simulink model "LQR_control_2019b"  (R2021a)
settings: Solver=VariableStepAuto  StartTime=0.0  StopTime=10.0  RelTol=1e-3
undefined symbols (not defined in the file or in its folder): HIL, K_lqr, qc_get_step_size, sigbuilder_block
libraries: simulink_extras x6, quarc_library x4, cstblocks x1
settings Model: Creator=AleFire  LastModifiedBy=arco
settings SolverCC: AlgebraicLoopSolver=TrustRegion
settings DebuggingCC: UnconnectedInputMsg=none  UnconnectedOutputMsg=none  UnconnectedLineMsg=none
settings ModelReferenceCC: EnableRefExpFcnMdlSchedulingChecks=off
settings RTWCC: Description=Generic Real-Time Target

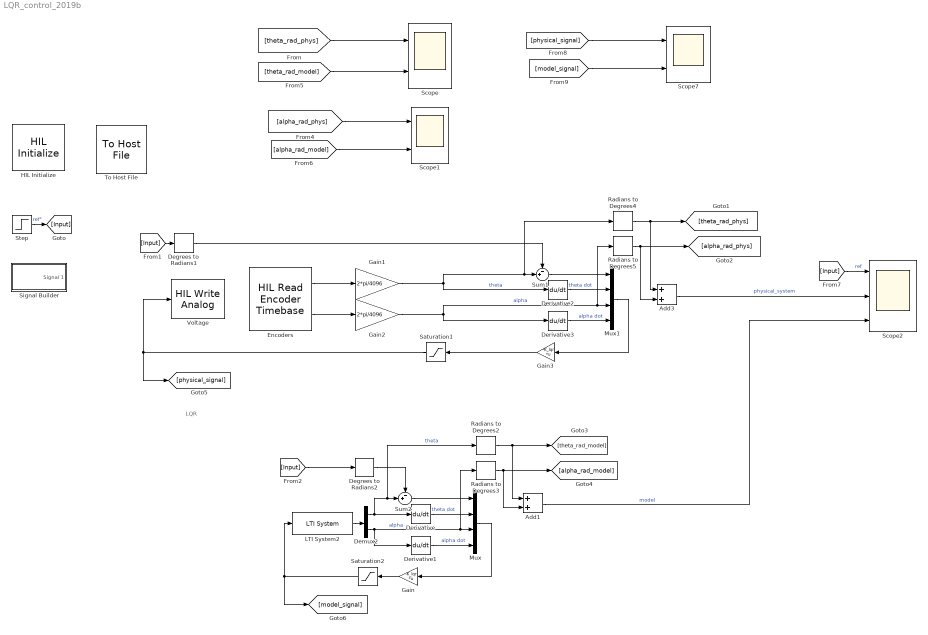
== system LQR_control_2019b ==
  note: LQR
  Add1 : Sum
  Add3 : Sum
  Degrees to Radians1 : simulink_extras/Transformations/Degrees to Radians
  Degrees to Radians2 : simulink_extras/Transformations/Degrees to Radians
  Demux2 : Demux  Outputs=2
  Derivative{,1..3} (4 alike) : Derivative
  Encoders : quarc_library/Data Acquisition/Generic/Timebases/HIL Read Encoder Timebase  object_name=HIL-1  clock=0  channels=[0:1]  samples_in_buffer=max(ceil(1/qc_get_step_size), 1)  active=on  vector_output=off  data_type_mode=Inherit via back propagation  data_type=double
  Gain : Gain  Gain=-K_lqr  Multiplication=Matrix(K*u)
  Gain1 : Gain  Gain=2*pi/4096
  Gain2 : Gain  Gain=2*pi/4096
  Gain3 : Gain  Gain=-K_lqr  Multiplication=Matrix(K*u)
  HIL Initialize : quarc_library/Data Acquisition/Generic/Configuration/HIL Initialize  Priority=-99  object_name=HIL-1  board_type=q2_usb  board_number=0  board_options=d0=digital;d1=digital;led=auto;update_rate=normal;decimation=1  exclusive=off  active=off  hardware_clocks=[0]  clock_modes=[]  initial_clock_frequencies=[]  set_clock_params_at_start=off  set_clock_params_at_switch_in=off  set_clock_frequencies_at_start=off  set_clock_frequencies_at_switch_in=off  analog_input_channels=[0:1]  analog_input_configurations=[]  analog_input_maximums=10  analog_input_minimums=-10  set_analog_input_params_at_start=on  set_analog_input_params_at_switch_in=off  analog_output_channels=[0:1]  analog_output_maximums=10  analog_output_minimums=-10  initial_analog_outputs=[0]  final_analog_outputs=[0]  watchdog_analog_outputs=0  set_analog_output_params_at_start=on  set_analog_output_params_at_switch_in=off  set_analog_outputs_at_start=on  set_analog_outputs_at_switch_in=off  set_analog_outputs_at_terminate=on  set_analog_outputs_at_switch_out=off  set_analog_outputs_on_watchdog=off  digital_input_channels=[]  digital_output_channels=[]  digital_output_configuration=[]  initial_digital_outputs=[1]  final_digital_outputs=[1]  watchdog_digital_outputs=[1]  set_digital_output_params_at_start=off  set_digital_output_params_at_switch_in=off  set_digital_outputs_at_start=on  set_digital_outputs_at_switch_in=off  set_digital_outputs_at_terminate=on  set_digital_outputs_at_switch_out=off  set_digital_outputs_on_watchdog=off  encoder_channels=[0:1]  quadrature=[4]  encoder_filter_frequency=[]  initial_encoder_counts=[0]  set_encoder_params_at_start=on  set_encoder_params_at_switch_in=off  set_encoder_counts_at_start=on  set_encoder_counts_at_switch_in=off  pwm_channels=[]  pwm_modes=[0]  pwm_frequency=1/0.020  pwm_configuration=[]  pwm_alignment=[]  pwm_polarity=[]  pwm_leading_deadband=[]  pwm_trailing_deadband=[]  initial_pwm_outputs=[0]  final_pwm_outputs=[0]  watchdog_pwm_outputs=[0]  set_pwm_params_at_start=on  set_pwm_params_at_switch_in=off  set_pwm_outputs_at_start=on  set_pwm_outputs_at_switch_in=off  set_pwm_outputs_at_terminate=on  set_pwm_outputs_at_switch_out=off  set_pwm_outputs_on_watchdog=off  other_output_channels=[]  initial_other_outputs=[]  final_other_outputs=[]  watchdog_other_outputs=[]  set_other_outputs_at_start=off  set_other_outputs_at_switch_in=off  set_other_outputs_at_terminate=off  set_other_outputs_at_switch_out=off  set_other_outputs_on_watchdog=off
  LTI System2 : cstblocks/LTI System  sys=sysestc  IC=[]
  Mux : Mux
  Mux1 : Mux
  Radians to Degrees{2..5} (4 alike) : simulink_extras/Transformations/Radians to Degrees
  Saturation1 : Saturate  UpperLimit=4.5  LowerLimit=-4.5
  Saturation2 : Saturate  UpperLimit=4.5  LowerLimit=-4.5
  Scope : Scope  NumInputPorts=2
  Scope1 : Scope  NumInputPorts=2
  Scope2 : Scope  NumInputPorts=3
  Scope7 : Scope  NumInputPorts=2
  Signal Builder : Subsystem  Tag=STV Subsys  LoadFcn=sigbuilder_block('load');  StartFcn=sigbuilder_block('start');  StopFcn=sigbuilder_block('stop');  ClipboardFcn=sigbuilder_block('clipboard');  mask(Sigbuilder block){tuvar=[0:10]}
      mask help: Simulink:masks:SigbuilderBlock_MD
      mask init:
      | if ~strcmp(get_param(bdroot(gcbh),'SimulationStatus'),'stopped') tuvar = sigbuilder_block('maskInit'); end
      settings: CopyFcn=sigbuilder_block('copy');  DeleteFcn=sigbuilder_block('delete');  ModelCloseFcn=sigbuilder_block('modelClose');  PreSaveFcn=sigbuilder_block('preSave');  PauseFcn=sigbuilder_block('pause');  ContinueFcn=sigbuilder_block('continue');  NameChangeFcn=sigbuilder_block('namechange');  OpenFcn=sigbuilder_block('open',[437.6 199.2 550.4 400 ]);  CloseFcn=sigbuilder_block('close');
      mask Display: plot(0, 0, 100, 100,[2, 2, 32, 32, 2], [68, 8, 8, 68, 68],[32, 2], [38, 38], [32, 19, 2],[53, 60, 44], [32, 17, 17, 2],[16, 16, 31, 31]);txt = getActiveGroup(gcbh);text(2, 100, txt,'verticalAlignment', 'top');
  Step : Step  After=20  SampleTime=0
  Sum1 : Sum  Inputs=-+|
  Sum2 : Sum  Inputs=-+|
  To Host File : quarc_library/Sinks/To Host/To Host File  file_name=data_%{date}_%{time}.mat  variable_name=data_%{date}_%{time}  decimation=1  sample_time=0.002  file_format=MAT-file v.5  options=No header or footer  append=off  final_file_name=data_20-Mar-2023_17-30-44.mat  bitrate=2000000
  Voltage : quarc_library/Data Acquisition/Generic/Immediate I//O/HIL Write Analog  object_name=HIL-1  channels=0  sample_time=-1  active=off  vector_input=off
  wires:
  Add1/1 -> Scope2/3  "model"
  Mux/1 -> Gain/1
  Demux2/1 -> Radians to Degrees2/1, Sum2/2, Derivative/1  "theta"
  Radians to Degrees3/1 -> [alpha_rad_model], Add1/2
  LTI System2/1 -> Demux2/1
  Degrees to Radians2/1 -> Sum2/1
  Saturation2/1 -> [model_signal], LTI System2/1
  Derivative1/1 -> Mux/4  "alpha dot"
  Gain/1 -> Saturation2/1
  Radians to Degrees2/1 -> [theta_rad_model], Add1/1
  Derivative/1 -> Mux/2  "theta dot"
  Sum2/1 -> Mux/1
  Demux2/2 -> Derivative1/1, Radians to Degrees3/1, Mux/3  "alpha"
  [Input] -> Degrees to Radians2/1
  [model_signal] -> Scope7/2
  [physical_signal] -> Scope7/1
  Step/1 -> [Input]  "ref°"
  [alpha_rad_phys] -> Scope1/1
  [Input] -> Scope2/1  "ref"
  [alpha_rad_model] -> Scope1/2
  [theta_rad_model] -> Scope/2
  [theta_rad_phys] -> Scope/1
  [Input] -> Degrees to Radians1/1
  Sum1/1 -> Mux1/1
  Saturation1/1 -> Voltage/1, [physical_signal]
  Radians to Degrees4/1 -> [theta_rad_phys], Add3/1
  Gain3/1 -> Saturation1/1
  Derivative2/1 -> Mux1/2  "theta dot"
  Derivative3/1 -> Mux1/4  "alpha dot"
  Gain1/1 -> Derivative2/1, Radians to Degrees4/1, Sum1/2  "theta"
  Gain2/1 -> Radians to Degrees5/1, Mux1/3, Derivative3/1  "alpha"
  Radians to Degrees5/1 -> [alpha_rad_phys], Add3/2
  Mux1/1 -> Gain3/1
  Add3/1 -> Scope2/2  "physical_system"
  Degrees to Radians1/1 -> Sum1/1
  Encoders/1 -> Gain1/1
  Encoders/2 -> Gain2/1

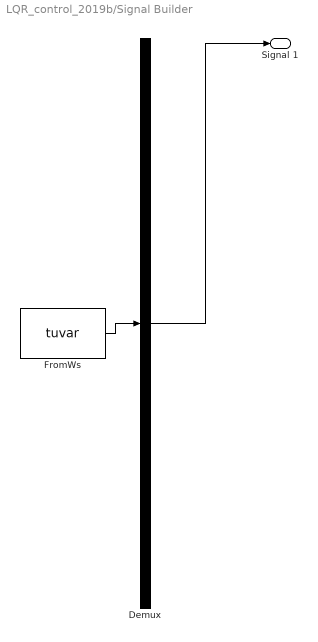
== system LQR_control_2019b/Signal Builder ==
  Demux : Demux  Tag=STV Demux  Outputs=1
      settings: DisplayOption=none
  FromWs : FromWorkspace  Tag=STV FromWs  VariableName=tuvar
      SigBuilderData=|
      | common.afterFinalStr = 'Extrapolate'
      | common.sampleTime = 0
      | dataSet.timeRange = [0 10]
      | dataSet.name = 'Group 1'
      | sbobj.Groups.Name = 'Group 1'
      | sbobj.Groups.Signals.Name = 'Signal 1'
      | sbobj.Groups.Signals.XData = [0 0.94 2 2 2.82 4 4 6 6 7.6 10]
      | sbobj.Groups.Signals.YData = [0 1.015 1.01 -0.285 0.83 0.125 0.665 0.785 -0.24 -0.325 0]
  Signal 1 : Outport  Tag=STV Outport
  wires:
  Demux/1 -> Signal 1/1
  FromWs/1 -> Demux/1
